simulink model "velocity_tracking"  (R2018b)
settings: Solver=ode8  StartTime=0.0  StopTime=14  FixedStep=0.05  RelTol=1e-3
settings Model: Creator=suvo.ganguli  LastModifiedBy=suvo.ganguli

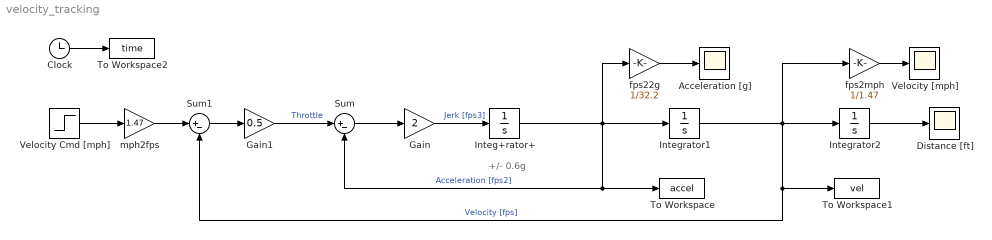
== system velocity_tracking ==
  note: +/- 0.6g
  Acceleration [g] : Scope
  Clock : Clock
  Distance [ft] : Scope
  Gain : Gain  Gain=2
  Gain1 : Gain  Gain=0.5
  Integ+rator+ : Integrator  LimitOutput=on  UpperSaturationLimit=0.6*32.2  LowerSaturationLimit=-0.6*32.2
  Integrator1 : Integrator  InitialCondition=20*1.47
  Integrator2 : Integrator
  Sum : Sum  Inputs=|+-
  Sum1 : Sum  Inputs=|+-
  To Workspace : ToWorkspace  VariableName=accel  SampleTime=-1
  To Workspace1 : ToWorkspace  VariableName=vel  SampleTime=-1
  To Workspace2 : ToWorkspace  VariableName=time  SampleTime=-1
  Velocity [mph] : Scope
  Velocity Cmd [mph] : Step  Time=0  Before=20  After=45  SampleTime=0
  fps22g : Gain  Gain=1/32.2
  fps2mph : Gain  Gain=1/1.47
  mph2fps : Gain  Gain=1.47
  wires:
  Sum/1 -> Gain/1
  Gain/1 -> Integ+rator+/1  "Jerk [fps3]"
  Integ+rator+/1 -> Integrator1/1, fps22g/1, To Workspace/1, Sum/2  "Acceleration [fps2]"
  Sum1/1 -> Gain1/1
  Integrator1/1 -> To Workspace1/1, Sum1/2, Integrator2/1, fps2mph/1  "Velocity [fps]"
  Gain1/1 -> Sum/1  "Throttle"
  Integrator2/1 -> Distance [ft]/1
  mph2fps/1 -> Sum1/1
  fps2mph/1 -> Velocity [mph]/1
  fps22g/1 -> Acceleration [g]/1
  Velocity Cmd [mph]/1 -> mph2fps/1
  Clock/1 -> To Workspace2/1
